simulink model "PLL_Simulering"  (R2020a)
settings: Solver=VariableStepAuto  StartTime=0  StopTime=0.5  RelTol=1e-3
InitFcn:
  | clear all;
libraries: powerlib x48, eePowerMeasurement x1, powerlib_meascontrol x1
(part 3 of 3)

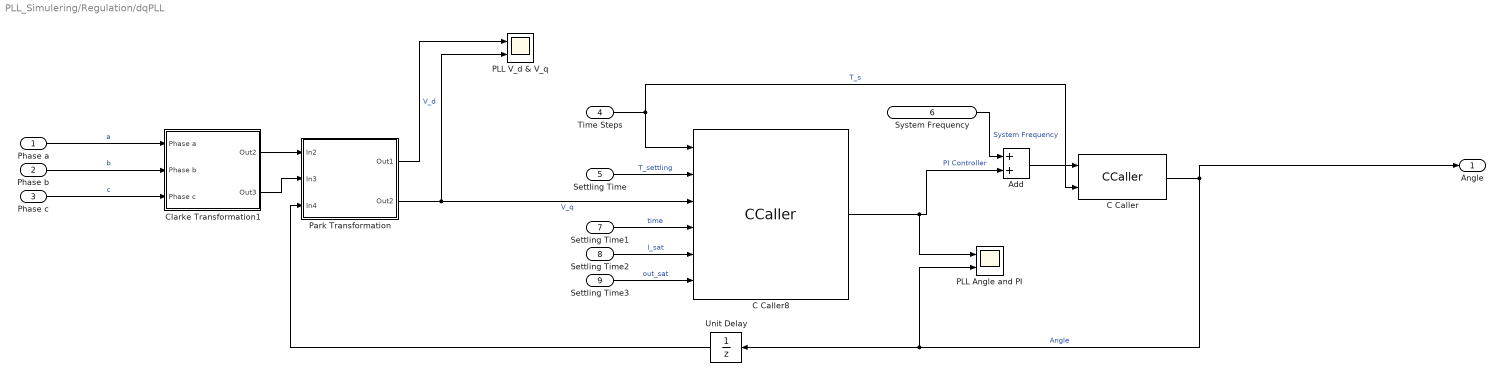
== system PLL_Simulering/Regulation/dqPLL ==
  Phase a : Inport
  Phase b : Inport  Port=2
  Phase c : Inport  Port=3
  Time Steps : Inport  Port=4
  Settling Time : Inport  Port=5
  System Frequency : Inport  Port=6
  Settling Time1 : Inport  Port=7
  Settling Time2 : Inport  Port=8
  Settling Time3 : Inport  Port=9
  Add : Sum  AccumDataTypeStr=double  OutDataTypeStr=double
  C Caller : CCaller  FunctionName=integrator  PortSpecificationStruct="%)30     .    : 4   8    (     @         %    \"     ,    !     0         %  0 \"0    $    _    07)G3F%M90  4&]R=$YA;64 4V-O<&4     26YD97@     5'EP90      4VEZ90      27-';&]B86P   X    P    !@    @    $          4    (     0    ,    !         !   P!O=70 #@   #     &    \"     0         !0    @    !     P    $         $  # &]U=  .    .     8    (    !          %    \"     $    &     0         0    !@   $]U='!U=   #@   #@    &    \"     8         !0    @    !     0    $         \"0    @               X    X    !@    @    $          4    (     0    8    !         !     &    9&]U8FQE   .    ,     8    (    !          %    \"     $    !     0         0  $ ,0    X    P    !@    @    ) @        4    (     0    $    !          (  0      #@   #@    &    \"     0         !0    @    !    !0    $         $     4   !E<G)O<@    X    X    !@    @    $          4    (     0    4    !         !     %    97)R;W(    .    .     8    (    !          %    \"     $    %     0         0    !0   $EN<'5T    #@   #@    &    \"     8         !0    @    !     0    $         \"0    @               X    X    !@    @    $          4    (     0    8    !         !     &    9&]U8FQE   .    ,     8    (    !          %    \"     $    !     0         0  $ ,0    X    P    !@    @    ) @        4    (     0    $    !          (  0      #@   #     &    \"     0         !0    @    !     P    $         $  # %1?<P .    ,     8    (    !          %    \"     $    #     0         0  , 5%]S  X    X    !@    @    $          4    (     0    4    !         !     %    26YP=70    .    .     8    (    !@         %    \"     $    !     0         )    \"            / _#@   #@    &    \"     0         !0    @    !    !@    $         $     8   !D;W5B;&4   X    P    !@    @    $          4    (     0    $    !         !   0 Q    #@   #     &    \"     D\"        !0    @    !     0    $          @ !"
  C Caller8 : CCaller  FunctionName=PID_Type_1  PortSpecificationStruct="%)30     .    * P   8    (     @         %    \"     <    !     0         %  0 \"0    $    _    07)G3F%M90  4&]R=$YA;64 4V-O<&4     26YD97@     5'EP90      4VEZ90      27-';&]B86P   X    P    !@    @    $          4    (     0    ,    !         !   P!O=70 #@   #     &    \"     0         !0    @    !     P    $         $  # &]U=  .    .     8    (    !          %    \"     $    &     0         0   ...(+3810 chars)"
  Clarke Transformation1 : Subsystem
  PLL Angle and PI : Scope  NumInputPorts=2
  PLL V_d & V_q : Scope  NumInputPorts=2
  Park Transformation : Subsystem
  Unit Delay : UnitDelay  SampleTime=-1  HasFrameUpgradeWarning=on
  Angle : Outport
  wires:
  Phase a/1 -> Clarke Transformation1/1(Phase a)  "a"
  Phase b/1 -> Clarke Transformation1/2(Phase b)  "b"
  Phase c/1 -> Clarke Transformation1/3(Phase c)  "c"
  Settling Time/1 -> C Caller8/2  "T_settling"
  System Frequency/1 -> Add/1  "System Frequency"
  Add/1 -> C Caller/1
  C Caller/1 -> Angle/1, PLL Angle and PI/2, Unit Delay/1  "Angle"
  Clarke Transformation1/1(Out2) -> Park Transformation/1(In2)
  Clarke Transformation1/2(Out3) -> Park Transformation/2(In3)
  Park Transformation/2(Out2) -> PLL V_d & V_q/2, C Caller8/3  "V_q"
  Unit Delay/1 -> Park Transformation/3(In4)
  Time Steps/1 -> C Caller/2, C Caller8/1  "T_s"
  C Caller8/1 -> PLL Angle and PI/1, Add/2  "PI Controller"
  Settling Time1/1 -> C Caller8/4  "time"
  Settling Time2/1 -> C Caller8/5  "I_sat"
  Settling Time3/1 -> C Caller8/6  "out_sat"
  Park Transformation/1(Out1) -> PLL V_d & V_q/1  "V_d"

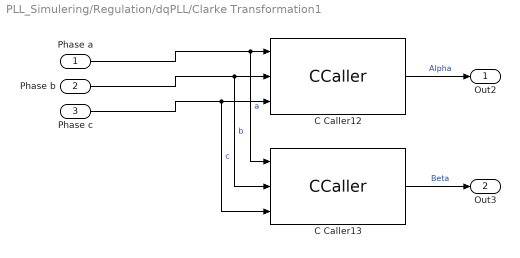
== system PLL_Simulering/Regulation/dqPLL/Clarke Transformation1 ==
  Phase a : Inport
  Phase b : Inport  Port=2
  Phase c : Inport  Port=3
  C Caller12 : CCaller  FunctionName=Clarke_alpha  PortSpecificationStruct="%)30     .    ^ 8   8    (     @         %    \"     0    !     0         %  0 \"0    $    _    07)G3F%M90  4&]R=$YA;64 4V-O<&4     26YD97@     5'EP90      4VEZ90      27-';&]B86P   X    P    !@    @    $          4    (     0    ,    !         !   P!O=70 #@   #     &    \"     0         !0    @    !     P    $         $  # &]U=  .    .     8    (    !          %    \"     $    &     0         0   ...(+2020 chars)"
  C Caller13 : CCaller  FunctionName=Clarke_beta  PortSpecificationStruct="%)30     .    ^ 8   8    (     @         %    \"     0    !     0         %  0 \"0    $    _    07)G3F%M90  4&]R=$YA;64 4V-O<&4     26YD97@     5'EP90      4VEZ90      27-';&]B86P   X    P    !@    @    $          4    (     0    ,    !         !   P!O=70 #@   #     &    \"     0         !0    @    !     P    $         $  # &]U=  .    .     8    (    !          %    \"     $    &     0         0   ...(+2020 chars)"
  Out2 : Outport
  Out3 : Outport  Port=2
  wires:
  Phase a/1 -> C Caller13/1, C Caller12/1  "a"
  Phase b/1 -> C Caller13/2, C Caller12/2  "b"
  Phase c/1 -> C Caller13/3, C Caller12/3  "c"
  C Caller12/1 -> Out2/1  "Alpha"
  C Caller13/1 -> Out3/1  "Beta"

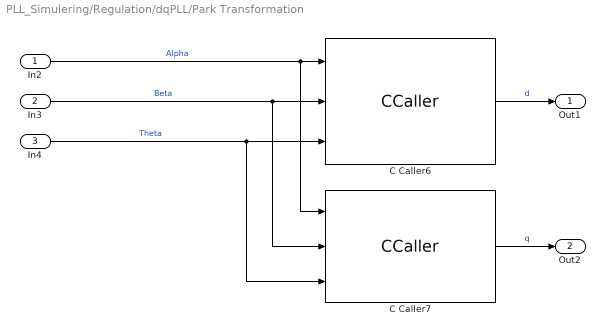
== system PLL_Simulering/Regulation/dqPLL/Park Transformation ==
  In2 : Inport
  In3 : Inport  Port=2
  In4 : Inport  Port=3
  C Caller6 : CCaller  FunctionName=Park_d  PortSpecificationStruct="%)30     .    * <   8    (     @         %    \"     0    !     0         %  0 \"0    $    _    07)G3F%M90  4&]R=$YA;64 4V-O<&4     26YD97@     5'EP90      4VEZ90      27-';&]B86P   X    P    !@    @    $          4    (     0    ,    !         !   P!O=70 #@   #     &    \"     0         !0    @    !     P    $         $  # &]U=  .    .     8    (    !          %    \"     $    &     0         0   ...(+2078 chars)"
  C Caller7 : CCaller  FunctionName=Park_q  PortSpecificationStruct="%)30     .    * <   8    (     @         %    \"     0    !     0         %  0 \"0    $    _    07)G3F%M90  4&]R=$YA;64 4V-O<&4     26YD97@     5'EP90      4VEZ90      27-';&]B86P   X    P    !@    @    $          4    (     0    ,    !         !   P!O=70 #@   #     &    \"     0         !0    @    !     P    $         $  # &]U=  .    .     8    (    !          %    \"     $    &     0         0   ...(+2078 chars)"
  Out1 : Outport
  Out2 : Outport  Port=2
  wires:
  In2/1 -> C Caller7/1, C Caller6/1  "Alpha"
  In3/1 -> C Caller7/2, C Caller6/2  "Beta"
  In4/1 -> C Caller7/3, C Caller6/3  "Theta"
  C Caller6/1 -> Out1/1  "d"
  C Caller7/1 -> Out2/1  "q"

== matlab function PLL_Simulering/Grid Source and Referance/MATLAB Function7 ==
  data: init_U_LL input; u_a_reff output; init_freq input; t input; u_b_reff output; u_c_reff output
function [u_a_reff, u_b_reff, u_c_reff] = positive_sequence(init_U_LL, init_freq, t)

omega_reff = init_freq * pi* 2;

varphi_reff = 0;


u_a_reff = sqrt(2/3)*init_U_LL*cos(omega_reff*t+varphi_reff);
u_b_reff = sqrt(2/3)*init_U_LL*cos(omega_reff*t+varphi_reff - (2/3)*pi);
u_c_reff = sqrt(2/3)*init_U_LL*cos(omega_reff*t+varphi_reff + (2/3)*pi);

end

== matlab function PLL_Simulering/Load & Cable Value Coeficients ==
  data: V_base_LL input; R_1 output; S_base_3 input; R_2 output; R_3 output; R_4 output; R_5 output; R_6 output; L_1 output; L_2 output; L_3 output; L_4 output; L_5 output; L_6 output
function [R_1, R_2, R_3, R_4, R_5, R_6, L_1, L_2, L_3, L_4, L_5, L_6] = GridConfigurationValues(V_base_LL, S_base_3)

Z_base = V_base_LL^2 / S_base_3;

R_1_base = 74.6e-3;
R_2_base = 74.6e-3;
R_3_base = 74.6e-3;
R_4_base = 74.6e-3;
R_5_base = 7.46e-3;

L_1_base = 2.375e-3;
L_2_base = 2.375e-3;
L_3_base = 2.375e-3;
L_4_base = 2.375e-3;
L_5_base = 0.237e-3;

R_1 = Z_base * R_1_base;
R_2 = Z_base * R_2_base;
R_3 = Z_base * R_3_base;
R_4 = Z_base * R_4_base;
R_5 = Z_base * R_5_base;
R_6 = Z_base * cos(26.6);

L_1 = Z_base * L_1_base;
L_2 = Z_base * L_2_base;
L_3 = Z_base * L_3_base;
L_4 = Z_base * L_4_base;
L_5 = Z_base * L_5_base;
L_6 = Z_base * sin(26.6);



end

== matlab function PLL_Simulering/Switch Control for Breakers ==
  data: senario input; S1 output; t input; S2 output; S3 output; S4 output; S5 output
function [S1, S2, S3, S4, S5]  = switch_control(senario, t)
S1 = 0;
S2 = 0;
S3 = 0;
S4 = 0;
S5 = 0;

if senario == 1
    S1 = 1;
    S2 = 1;
    S3 = 1;
    S4 = 0;
    S5 = 1;
        
elseif senario == 2
    S1 = 1;
    S2 = 1;
    S3 = 1;
    S4 = 0;
    S5 = 1;
    
elseif senario == 3
    S1 = 1;
    S2 = 1;
    S3 = 1;
    S4 = 0;
    S5 = 1;
  
elseif senario == 4
    S1 = 1;
    S2 = 1;
    S3 = 1;
    S4 = 0;
    S5 = 1;
       
elseif senario == 5
    S1 = 1;
    S2 = 1;
    S3 = 1;
    S4 = 0;
    S5 = 1;    
    
elseif senario == 6
    S1 = 1;
    S2 = 1;
    S3 = 1;
    S4 = 0;
    S5 = 1;
    
elseif senario == 7
    if 3 <= t
        S1 =0;
        S2 =0;
        S3 =1;
        S4 =0;
        S5 =1;
    elseif 1 <= t
        S1 =0;
        S2 =1;
        S3 =1;
        S4 =0;
        S5 =1;
    elseif t < 1
        S1 =1;
        S2 =1;
        S3 =1;
        S4 =0;
        S5 =1;
    end
    
elseif senario == 8
    if 1 <= t
        S1 =1;
        S2 =1;
        S3 =1;
        S4 =0;
        S5 =0;
    elseif t < 1
        S1 =1;
        S2 =1;
        S3 =1;
        S4 =0;
        S5 =1;
    
    end

else
    
end

end

== matlab function PLL_Simulering/Grid Source and Referance/MATLAB Function1 ==
  data: U_LL1 input; u_a1 output; omega_1 input; varphi_1 input; t input; u_b1 output; u_c1 output
function [u_a1, u_b1, u_c1] = positive_sequence(U_LL1, omega_1, varphi_1, t)



u_a1 = sqrt(2/3)*U_LL1*cos(omega_1*t+varphi_1);
u_b1 = sqrt(2/3)*U_LL1*cos(omega_1*t+varphi_1 - (2/3)*pi);
u_c1 = sqrt(2/3)*U_LL1*cos(omega_1*t+varphi_1 + (2/3)*pi);

end

== matlab function PLL_Simulering/Grid Source and Referance/MATLAB Function3 ==
  data: U_LL3 input; u_a3 output; omega_3 input; varphi_3 input; t input; u_b3 output; u_c3 output
function [u_a3, u_b3, u_c3] = harmonic_oscillation(U_LL3, omega_3, varphi_3, t)

u_a3 = sqrt(2/3)*U_LL3*cos(omega_3*t+varphi_3);
u_b3 = sqrt(2/3)*U_LL3*cos(omega_3*t+varphi_3 - (2/3)*pi);
u_c3 = sqrt(2/3)*U_LL3*cos(omega_3*t+varphi_3 + (2/3)*pi);

end

== matlab function PLL_Simulering/Grid Source and Referance/MATLAB Function2 ==
  data: U_LL2 input; u_a2 output; omega_2 input; varphi_2 input; t input; u_b2 output; u_c2 output
function [u_a2, u_b2, u_c2] = negative_sequence(U_LL2, omega_2, varphi_2, t)

u_a2 = sqrt(2/3)*U_LL2*cos(omega_2*t+varphi_2);
u_b2 = sqrt(2/3)*U_LL2*cos(omega_2*t+varphi_2 + (2/3)*pi);
u_c2 = sqrt(2/3)*U_LL2*cos(omega_2*t+varphi_2 - (2/3)*pi);

end

== matlab function PLL_Simulering/Grid Source and Referance/MATLAB Function ==
  data: senario input; U_LL1 output; t input; omega_1 output; varphi_1 output; init_freq input; init_U_LL1 input
function [U_LL1, omega_1, varphi_1]  = positive_sequence_senario_variables(senario, t, init_freq, init_U_LL1)

U_LL1 = init_U_LL1;
omega_1 = 2*pi*init_freq;
varphi_1 = 0;

if senario == 1
    U_LL1 = init_U_LL1;
    omega_1 = 2*pi*init_freq;
    
    if 7 <= t
        varphi_1 = 0;
    elseif 5 <= t
        varphi_1 = -30;
    elseif 3 <= t
        varphi_1 = -40;
    elseif 1 <= t
        varphi_1 = -10; 
    elseif t < 1
        varphi_1 = 0;
    end
        
end    
if senario == 2
    U_LL1 = init_U_LL1;
    
% Change in Frequency
    if 11.5 <= t
        omega_1 = 2*pi*init_freq;
        
    elseif (11 <= t) && (t <= 11.5)
        new_freq = (init_freq - 1) + (t - 11)*2;
        omega_1 = 2*pi*new_freq;
        
    elseif 7.5 < t
        new_freq = init_freq - 1;
        omega_1 = 2*pi*new_freq;
        
    elseif (7 <= t) && (t <= 7.5)
        new_freq = init_freq - (t - 7)*2;
        omega_1 = 2*pi*new_freq;
        
    elseif 4.5 <= t
        new_freq = init_freq;
        omega_1 = 2*pi*new_freq;
        
    elseif (4 <= t) && (t <= 4.5)
        new_freq = (init_freq + 1) - (t - 4)*2;
        omega_1 = 2*pi*new_freq;
        
    elseif 1.5 <= t
        new_freq = init_freq + 1;
        omega_1 = 2*pi*new_freq;
        
    elseif (1 <= t) && (t <= 1.5)
        new_freq = init_freq + (t - 1)*2;
        omega_1 = 2*pi*new_freq;
        
    elseif t <= 1
        omega_1 = 2*pi*init_freq;
        
    end
    
% Change in Phase Angle
    if 11 <= t
        varphi_1 = 0;
    elseif 7 <= t
        varphi_1 = -30;
    elseif 4 <= t   
        varphi_1 = 0;
    elseif 1 <= t
        varphi_1 = 30;
    elseif t < 1
        varphi_1 = 0;
    end
end    
if senario == 3
    omega_1 = 2*pi*init_freq;
    varphi_1 = 0;
    
% Change in U_LL
    if 15 <= t
        U_LL1 = init_U_LL1;
    elseif 13 <= t
        U_LL1 = init_U_LL1*1.1;
    elseif 11 <= t   
        U_LL1 = init_U_LL1;
    elseif 9 <= t
        U_LL1 = init_U_LL1 *1.05;
    elseif 7 <= t
        U_LL1 = init_U_LL1;
    elseif 5 <= t
        U_LL1 = init_U_LL1 *0.9;
    elseif 3 <= t   
        U_LL1 = init_U_LL1;
    elseif 1 <= t
        U_LL1 = init_U_LL1 * 0.95;
    elseif t < 1
        U_LL1 = init_U_LL1;
    end
end    
if senario == 4
    U_LL1 = init_U_LL1;
    omega_1 = 2*pi*init_freq;
    varphi_1 = 0;
end    
if senario == 5
    U_LL1 = init_U_LL1;
    omega_1 = 2*pi*init_freq;
    varphi_1 = 0;
end    
if senario == 6
    U_LL1 = init_U_LL1;
    omega_1 = 2*pi*init_freq;
    varphi_1 = 0;
end    
if senario == 7
    U_LL1 = init_U_LL1;
    omega_1 = 2*pi*init_freq;
    varphi_1 = 0;
end    
if senario == 8
    U_LL1 = init_U_LL1;
    omega_1 = 2*pi*init_freq;
    varphi_1 = 0;
    
end

end

== matlab function PLL_Simulering/Grid Source and Referance/MATLAB Function4 ==
  data: senario input; U_LL2 output; t input; omega_2 output; varphi_2 output; init_freq input; init_U_LL2 input
function [U_LL2, omega_2, varphi_2]  = positive_sequence_senario_variables(senario, t, init_freq, init_U_LL2)
U_LL2 = init_U_LL2;
omega_2 = 2*pi*init_freq;
varphi_2 = 0;

if senario == 1
    U_LL2 = 0;
    omega_2 = 2*pi*0;
    varphi_2 = 0;
end   
if senario == 2
    U_LL2 = 0;
    omega_2 = 2*pi*0;
    varphi_2 = 0;
end    
if senario == 3
    U_LL2 = 0;
    omega_2 = 2*pi*0;
    varphi_2 = 0;
end  
if senario == 4
    new_freq = init_freq * -1;
    omega_2 = 2*pi*new_freq;
    varphi_2 = 0;
    
    if 1 <= t
        U_LL2 = init_U_LL2 *0.02;
    elseif t < 1
        U_LL2 = 0;
    end
end       
if senario == 5
    varphi_2 = 0;
    
    if 8 <= t
        new_freq = init_freq * 0;
        omega_2 = 2*pi*new_freq;
        U_LL2 = init_U_LL2 * 0;
    elseif 7 <= t
        new_freq = init_freq * 31;
        omega_2 = 2*pi*new_freq;
        U_LL2 = init_U_LL2 * 0.02;
    elseif 6 <= t
        new_freq = init_freq * 0;
        omega_2 = 2*pi*new_freq;
        U_LL2 = init_U_LL2 * 0;
    elseif 5 <= t
        new_freq = init_freq * 19;
        omega_2 = 2*pi*new_freq;
        U_LL2 = init_U_LL2 * 0.02;
    elseif 4 <= t
        new_freq = init_freq * 0;
        omega_2 = 2*pi*new_freq;
        U_LL2 = init_U_LL2 * 0;
    elseif 3 <= t
        new_freq = init_freq * -5;
        omega_2 = 2*pi*new_freq;
        U_LL2 = init_U_LL2 * 0.02;
    elseif 2 <= t
        new_freq = init_freq * 0;
        omega_2 = 2*pi*new_freq;
        U_LL2 = init_U_LL2 * 0;
    elseif 1 <= t
        new_freq = init_freq * 2;
        omega_2 = 2*pi*new_freq;
        U_LL2 = init_U_LL2 * 0.02;
    elseif t < 1
        new_freq = init_freq * 0;
        omega_2 = 2*pi*new_freq;
        U_LL2 = init_U_LL2 * 0;  
    end
end   
if senario == 6
    varphi_2 = 0;
    
    if 21 <= t
        new_freq = init_freq / (50/15.9);
        omega_2 = 2*pi*new_freq;
        U_LL2 = init_U_LL2 * 0.02;
    elseif 16 <= t
        new_freq = 0;
        omega_2 = 2*pi*new_freq;
        U_LL2 = init_U_LL2 * 0;
    elseif 11 <= t
        new_freq = init_freq / 5;
        omega_2 = 2*pi*new_freq;
        U_LL2 = init_U_LL2 * 0.02;
    elseif 6 <= t
        new_freq = 0;
        omega_2 = 2*pi*new_freq;
        U_LL2 = init_U_LL2 * 0;
    elseif 1 <= t
        new_freq = init_freq / 10;
        omega_2 = 2*pi*new_freq;
        U_LL2 = init_U_LL2 * 0.02;
    elseif t < 1
        new_freq = init_freq * 0;
        omega_2 = 2*pi*new_freq;
        U_LL2 = init_U_LL2 * 0;
    end
end  
if senario == 7
    new_freq = init_freq * 0;
    omega_2 = 2*pi*new_freq * 0;
    U_LL2 = init_U_LL2 * 0;
    varphi_2 = 0;
end   
if senario == 8
    new_freq = init_freq * 0;
    omega_2 = 2*pi*new_freq * 0;
    U_LL2 = init_U_LL2 * 0;
    varphi_2 = 0; 
end
    
end

== matlab function PLL_Simulering/Grid Source and Referance/MATLAB Function5 ==
  data: senario input; U_LL3 output; t input; omega_3 output; varphi_3 output; init_freq input; init_U_LL3 input
function [U_LL3, omega_3, varphi_3]  = harmonic_oscillation(senario, t, init_freq, init_U_LL3)
U_LL3 = init_U_LL3;
omega_3 = 2*pi*init_freq;
varphi_3 = 0;

if senario == 1
    U_LL3 = 0;
    omega_3 = 2*pi*0;
    varphi_3 = 0;
end
if senario == 2
    U_LL3 = 0;
    omega_3 = 2*pi*0;
    varphi_3 = 0;
end    
if senario == 3
    U_LL3 = 0;
    omega_3 = 2*pi*0;
    varphi_3 = 0;
end  
if senario == 4
    U_LL3 = 0;
    omega_3 = 2*pi*0;
    varphi_3 = 0;
end      
if senario == 5
    varphi_3 = 0;
   
% Change of frequency
    if 4 <= t
        new_freq = 0;
        omega_3 = 2*pi*new_freq;
        varphi_3 = 0;
    elseif 3 <= t
        new_freq = init_freq * 7;
        omega_3 = 2*pi*new_freq;
        varphi_3 = 0;
    elseif t < 3
    new_freq = 0;
    omega_3 = 2*pi*new_freq;
    end
    
% Change of U_LL
    if 4 <= t
        U_LL3 = 0;
    elseif 3 <= t
        U_LL3 = init_U_LL3*0.02;
    elseif t < 3
        U_LL3 = 0;
    end
end    
if senario == 6
    U_LL3 = 0;
    omega_3 = 2*pi*0;
    varphi_3 = 0;
end    
if senario == 7
    U_LL3 = 0;
    omega_3 = 2*pi*0;
    varphi_3 = 0;
end    
if senario == 8
    U_LL3 = 0;
    omega_3 = 2*pi*0;
    varphi_3 = 0;
end


end

== matlab function PLL_Simulering/Filter Value Coeficients ==
  data: f input; L_1 output; f_sw input; U_LL input; S_base input; Mi input; L_2 output; R_f output; C_f output; V_DC output; f_res output
function [L_1, L_2, R_f, C_f, V_DC, f_res]= FilterConfigurationValues(f, f_sw, U_LL, S_base, Mi)

Z_b = U_LL^2/S_base;

%omega_b = 2*pi*f;
%C_b = 1 / (omega_b*Z_b);
%V_DC = (2*U_LL*sqrt(2))/ (Mi*sqrt(3));
%I_max_delta = (S_base / sqrt(3)*U_LL)*1.1;
%L_1 = V_DC/ (6*f_sw*I_max_delta);
%C_f = 0.05 * C_b;
%omega_sw = 2*pi*f_sw;
%L_2 = 6 / (C_f*omega_sw);
%omega_res = sqrt((L_1 + L_2)/(L_1*L_2*C_f));
%f_res = 1/(2*pi)*omega_res;
%R_f = 1 / (3*C_f*omega_res);

L_1 = Z_b*0.071;
L_2 = Z_b*0.043;
C_f = Z_b*0.068;

V_DC = (2*U_LL*sqrt(2))/ (Mi*sqrt(3));
omega_res = sqrt((L_1 + L_2)/(L_1*L_2*C_f));
f_res = 1/(2*pi)*omega_res;
R_f = 1 / (3*C_f*omega_res);



end
